simulink library "MedusaPremix"  (R2022b)
settings: Solver=VariableStepAuto  StartTime=0.0  StopTime=10.0  RelTol=1e-3
values from neighbouring files (symbols this model uses):
  PremixConfig = struct('sample_rate_in_hertz', sample_rate_in_hertz,                            'frame_size', frame_size,                            'rgain_SILENT_GAIN', rgain_SILENT_GAIN,                            'granularity', internal_granularity,                            'LR_in', LR_in, 'LR_out', LR_out,                            'CS_in', CS_in, 'CS_out', CS_out,                            'NumCenterOut' ...(+550 chars)    [MedusaPremixInit.m]
  PremixTune = MedusaPremixTuneInit(tuneFileName, headrestTuneFileName, overheadTuneFileName, MedusaParams)    [MedusaPremixInit.m]    (also in MedusaPremixTuneInit.m = load(tuneFileName))
undefined symbols (not defined in the file or in its folder): carModel, mode, MSConfig, Row
libraries: TuneVar x286, TOP x202, dspmtrx3 x146, FeaturePath x86, matrix_library x20, PooliirLib x8, Pooliir x4
(part 1 of 22)
settings Model: Creator=jk1043656  LastModifiedBy=fz1054048
settings SolverCC: AlgebraicLoopSolver=TrustRegion
settings DataIOCC: ReturnWorkspaceOutputs=off
settings DebuggingCC: UnconnectedInputMsg=warning  UnconnectedOutputMsg=warning  UnconnectedLineMsg=warning  SFMachineParentedDataDiag=warning  ArithmeticOperatorsInVariantConditions=warning
settings ModelReferenceCC: EnableRefExpFcnMdlSchedulingChecks=on
settings SFSimCC: CustomCodeUndefinedFunction=UseInterfaceOnly

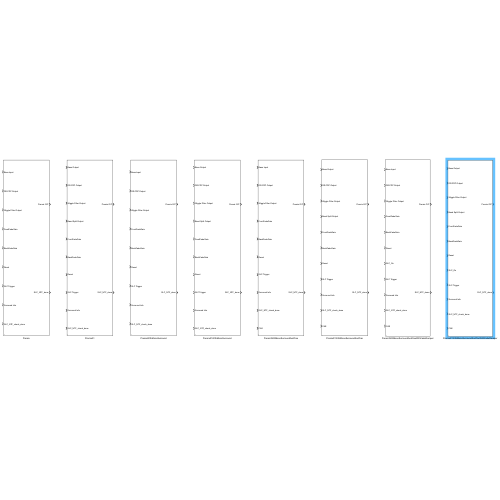
[thumbnail: Simulink's stored preview of the top-level diagram]
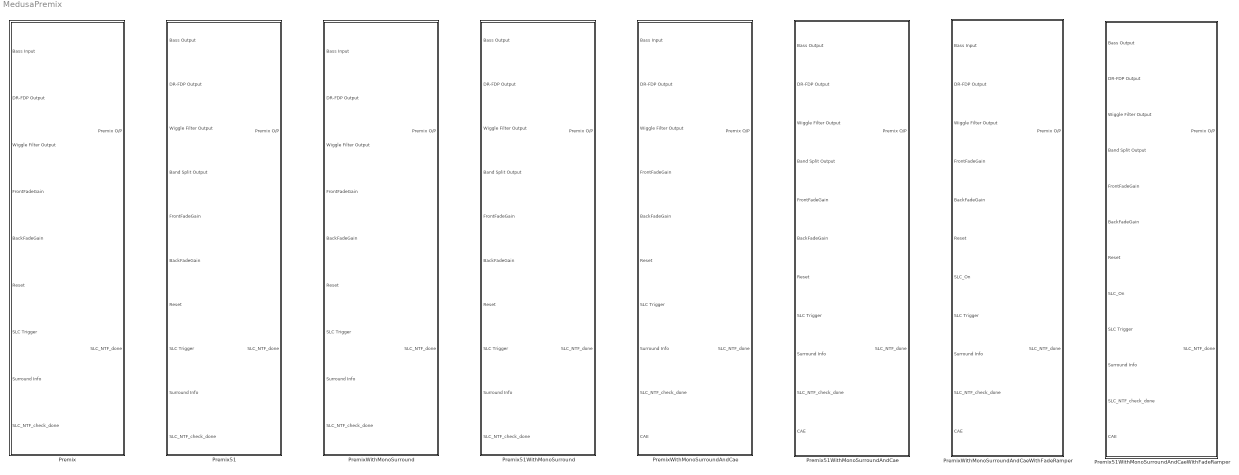
== system MedusaPremix ==
  Premix : Subsystem  mask(Medusa Premix 5H){MedusaPremixConfig=PremixConfig, MedusaPremixTune=PremixTune}
      mask prompts: MedusaPremixConfig "Config struct name:"; MedusaPremixTune "Tune struct name:"
      mask init:
      | % RTC_SIM_OBJ = RTC_SimData();
      | 
      | % MedusaConfig = generateMedusaConfig(system_definitions);
      | 
      | % Initialize model parameters
      | % MedusaPremixExampleInit(MedusaConfig);
  Premix51 : Subsystem  mask{MedusaPremixConfig=PremixConfig, MedusaPremixTune=PremixTune}
      mask prompts: MedusaPremixConfig "Config Struct Name"; MedusaPremixTune "Tune Struct Name"
      mask init:
      | % RTC_SIM_OBJ = RTC_SimData();
      | 
      | % MedusaConfig = generateMedusaConfig(system_definitions);
      | 
      | % Initialize model parameters
      | % MedusaPremixExampleInit(MedusaConfig);
  Premix51WithMonoSurround : Subsystem  mask{MedusaPremixConfig=PremixConfig, MedusaPremixTune=PremixTune, MSConfig=MSConfig}
      mask prompts: MedusaPremixConfig "Config Struct Name"; MedusaPremixTune "Tune Struct Name"; MSConfig "Mono-Surround Config"
      mask init:
      | % RTC_SIM_OBJ = RTC_SimData();
      | 
      | % MedusaConfig = generateMedusaConfig(system_definitions);
      | 
      | % Initialize model parameters
      | % MedusaPremixExampleInit(MedusaConfig);
  Premix51WithMonoSurroundAndCae : Subsystem  mask(Medusa Premix 5H){MedusaPremixConfig=PremixConfig, MedusaPremixTune=PremixTune, MSConfig=MSConfig}
      mask prompts: MedusaPremixConfig "Config struct name:"; MedusaPremixTune "Tune struct name:"; MSConfig "Mono-Surround Config:"
      mask init:
      | % RTC_SIM_OBJ = RTC_SimData();
      | 
      | % MedusaConfig = generateMedusaConfig(system_definitions);
      | 
      | % Initialize model parameters
      | % MedusaPremixExampleInit(MedusaConfig);
  Premix51WithMonoSurroundAndCaeWithFadeRamper : Subsystem  AncestorBlock=MedusaPremix/Premix 5.1 with Mono-Surround & CAE with Fade Ramper  mask(Medusa Premix 5H){MedusaPremixConfig=PremixConfig, MedusaPremixTune=PremixTune, MSConfig=MSConfig}
      mask prompts: MedusaPremixConfig "Config struct name:"; MedusaPremixTune "Tune struct name:"; MSConfig "Mono-Surround Config:"
      mask init:
      | % RTC_SIM_OBJ = RTC_SimData();
      | 
      | % MedusaConfig = generateMedusaConfig(system_definitions);
      | 
      | % Initialize model parameters
      | % MedusaPremixExampleInit(MedusaConfig);
      settings: LibrarySourceBlock=MedusaPremix/Premix 5.1 with Mono-Surround & CAE with Fade Ramper
  PremixWithMonoSurround : Subsystem  mask(Medusa Premix 5H){MedusaPremixConfig=PremixConfig, MedusaPremixTune=PremixTune, MSConfig=MSConfig}
      mask prompts: MedusaPremixConfig "Config struct name:"; MedusaPremixTune "Tune struct name:"; MSConfig "Mono-Surround Config:"
      mask init:
      | % RTC_SIM_OBJ = RTC_SimData();
      | 
      | % MedusaConfig = generateMedusaConfig(system_definitions);
      | 
      | % Initialize model parameters
      | % MedusaPremixExampleInit(MedusaConfig);
  PremixWithMonoSurroundAndCae : Subsystem  mask(Medusa Premix 5H){MedusaPremixConfig=PremixConfig, MedusaPremixTune=PremixTune, MSConfig=MSConfig}
      mask prompts: MedusaPremixConfig "Config struct name:"; MedusaPremixTune "Tune struct name:"; MSConfig "Mono-Surround Config:"
      mask init:
      | % RTC_SIM_OBJ = RTC_SimData();
      | 
      | % MedusaConfig = generateMedusaConfig(system_definitions);
      | 
      | % Initialize model parameters
      | % MedusaPremixExampleInit(MedusaConfig);
  PremixWithMonoSurroundAndCaeWithFadeRamper : Subsystem  AncestorBlock=MedusaPremix/Premix with Mono-Surround & CAE with Fade Ramper  mask(Medusa Premix 5H){MedusaPremixConfig=PremixConfig, MedusaPremixTune=PremixTune, MSConfig=MSConfig}
      mask prompts: MedusaPremixConfig "Config struct name:"; MedusaPremixTune "Tune struct name:"; MSConfig "Mono-Surround Config:"
      mask init:
      | % RTC_SIM_OBJ = RTC_SimData();
      | 
      | % MedusaConfig = generateMedusaConfig(system_definitions);
      | 
      | % Initialize model parameters
      | % MedusaPremixExampleInit(MedusaConfig);
      settings: LibrarySourceBlock=MedusaPremix/Premix with Mono-Surround & CAE with Fade Ramper

== system MedusaPremix/Premix ==
  Bass Input : Inport
  DR-FDP Output : Inport  Port=2
  Wiggle Filter Output : Inport  Port=3
  FrontFadeGain : Inport  Port=4
  BackFadeGain : Inport  Port=5
  Reset : Inport  Port=6
  SLC Trigger : Inport  Port=7
  Surround Info : Inport  Port=8
  SLC_NTF_check_done : Inport  Port=9
  Fade Inputs : Subsystem
  Fade Tuning : Subsystem
  FeaturePath : FeaturePath/FeaturePath  FeatureName=Premix  IsGroup=off  GroupNumber=-1  DeclarePackages=off  PackageNames=mode,carModel  IsToolGroup=off  TriggerInit=[145 479 260 586]
      settings: SourceProductName=Bose Talaria
  Full Mixing Matrix_Center Surround : Subsystem
  Full Mixing Matrix_Left : Subsystem
  Full Mixing Matrix_Right : Subsystem
  Function-Call Split : FunctionCallSplit  IconShape=distinctive  NumOutputPorts=3  OutputPortLayout=default
  Function-Call Split1 : FunctionCallSplit  IconShape=distinctive  NumOutputPorts=3  OutputPortLayout=default
  Input Organizer : Subsystem
  Matrix Concatenate : Concatenate  NumInputs=3  Mode=Multidimensional array  ConcatenateDimension=2
  Merge NTF_done : Subsystem
  SLC Tuning : Subsystem
  Split NTF_check_done : MATLAB Function  TreatAsAtomicUnit=on
  Premix O/P : Outport  VectorParamsAs1DForOutWhenUnconnected=off
  SLC_NTF_done : Outport  Port=2  VectorParamsAs1DForOutWhenUnconnected=off
  wires:
  Wiggle Filter Output/1 -> Input Organizer/3(WF O/P)
  Fade Inputs/2(triggerCS) -> Full Mixing Matrix_Center Surround/7(Fade Request Trigger)
  [Left_Output] -> Matrix Concatenate/2
  Function-Call Split1/2 -> Full Mixing Matrix_Center Surround/3(SLC Request Trigger)
  Function-Call Split/3 -> Full Mixing Matrix_Right/2(RST Trigger)
  Fade Inputs/5(BackFadeGain) -> Full Mixing Matrix_Left/9(Back Fade Gain), Full Mixing Matrix_Center Surround/9(Back Fade Gain), Full Mixing Matrix_Right/9(Back Fade Gain)
  Input Organizer/3(Left Channel Inputs) -> Full Mixing Matrix_Left/1(Audio Channel Inputs)
  Full Mixing Matrix_Left/1(Output) -> [Left_Output]
  Fade Inputs/1(triggerLeft) -> Full Mixing Matrix_Left/7(Fade Request Trigger)
  Full Mixing Matrix_Left/2(SLC_NTF_done) -> Merge NTF_done/1(SLC_NTF_done_Left)
  Fade Inputs/4(FrontFadeGain) -> Full Mixing Matrix_Left/8(Front Fade Gain), Full Mixing Matrix_Center Surround/8(Front Fade Gain), Full Mixing Matrix_Right/8(Front Fade Gain)
  Full Mixing Matrix_Right/2(SLC_NTF_done) -> Merge NTF_done/3(SLC_NTF_done_Right)
  Function-Call Split1/1 -> Full Mixing Matrix_Left/3(SLC Request Trigger)
  Surround Info/1 -> Full Mixing Matrix_Right/4(SLC In), Full Mixing Matrix_Center Surround/4(SLC In), Full Mixing Matrix_Left/4(SLC In)
  Split NTF_check_done/4(fcncall_AND()) -> Merge NTF_done/Trigger
  SLC Trigger/1 -> Function-Call Split1/1
  Input Organizer/1(Right Channel Inputs) -> Full Mixing Matrix_Right/1(Audio Channel Inputs)
  Function-Call Split/2 -> Full Mixing Matrix_Center Surround/2(RST Trigger)
  Input Organizer/2(CS Channel Inputs) -> Full Mixing Matrix_Center Surround/1(Audio Channel Inputs)
  Bass Input/1 -> Input Organizer/1(Bass O/P)
  Function-Call Split/1 -> Full Mixing Matrix_Left/2(RST Trigger)
  Reset/1 -> Function-Call Split/1
  Split NTF_check_done/1(fcncall_Left()) -> Full Mixing Matrix_Left/5(SLC_NTF_check_done)
  [CS_Output] -> Matrix Concatenate/1
  SLC_NTF_check_done/1 -> Split NTF_check_done/Trigger
  [Right_Output] -> Matrix Concatenate/3
  Full Mixing Matrix_Center Surround/1(Output) -> [CS_Output]
  BackFadeGain/1 -> Fade Inputs/2(BackGain)
  Split NTF_check_done/2(fcncall_CS()) -> Full Mixing Matrix_Center Surround/5(SLC_NTF_check_done)
  Matrix Concatenate/1 -> Premix O/P/1
  SLC Tuning/1(SLC Tune Out) -> Full Mixing Matrix_Left/6(SLC Tune In), Full Mixing Matrix_Center Surround/6(SLC Tune In), Full Mixing Matrix_Right/6(SLC Tune In)
  Full Mixing Matrix_Center Surround/2(SLC_NTF_done) -> Merge NTF_done/2(SLC_NTF_done_CS)
  Fade Inputs/3(triggerRight) -> Full Mixing Matrix_Right/7(Fade Request Trigger)
  Merge NTF_done/1(SLC_NTF_done) -> SLC_NTF_done/1
  FrontFadeGain/1 -> Fade Inputs/1(FrontGain)
  Split NTF_check_done/3(fcncall_Right()) -> Full Mixing Matrix_Right/5(SLC_NTF_check_done)
  Fade Tuning/1(Fade Tune Out) -> Full Mixing Matrix_Left/10(Fade Tune In), Full Mixing Matrix_Center Surround/10(Fade Tune In), Full Mixing Matrix_Right/10(Fade Tune In)
  Full Mixing Matrix_Right/1(Output) -> [Right_Output]
  DR-FDP Output/1 -> Input Organizer/2(DR-FDP O/P)
  Function-Call Split1/3 -> Full Mixing Matrix_Right/3(SLC Request Trigger)

== system MedusaPremix/Premix51 ==
  Bass Output : Inport
  DR-FDP Output : Inport  Port=2
  Wiggle Filter Output : Inport  Port=3
  Band Split Output : Inport  Port=4
  FrontFadeGain : Inport  Port=5
  BackFadeGain : Inport  Port=6
  Reset : Inport  Port=7
  SLC Trigger : Inport  Port=8
  Surround Info : Inport  Port=9
  SLC_NTF_check_done : Inport  Port=10
  Fade Inputs : Subsystem
  Fade Tuning : Subsystem
  FeaturePath : FeaturePath/FeaturePath  FeatureName=Premix  IsGroup=off  GroupNumber=-1  DeclarePackages=off  PackageNames=mode,carModel  IsToolGroup=off  TriggerInit=[575 894 690 1001]
      settings: SourceProductName=Bose Talaria
  Full Mixing Matrix_Center Surround : Subsystem
  Full Mixing Matrix_Left : Subsystem
  Full Mixing Matrix_Right : Subsystem
  Function-Call Split : FunctionCallSplit  IconShape=distinctive  NumOutputPorts=3  OutputPortLayout=default
  Function-Call Split1 : FunctionCallSplit  IconShape=distinctive  NumOutputPorts=3  OutputPortLayout=default
  Input Organizer : Subsystem
  MATLAB Function : MATLAB Function  TreatAsAtomicUnit=on
  Matrix Concatenate : Concatenate  NumInputs=3  Mode=Multidimensional array  ConcatenateDimension=2
  Merge NTF_done : Subsystem
  SLC Tuning : Subsystem
  Premix O/P : Outport  VectorParamsAs1DForOutWhenUnconnected=off
  SLC_NTF_done : Outport  Port=2  VectorParamsAs1DForOutWhenUnconnected=off
  wires:
  Full Mixing Matrix_Right/1(Output) -> [Right_Output]
  Input Organizer/2(CS Channel Inputs) -> Full Mixing Matrix_Center Surround/1(Audio Channel Inputs)
  Function-Call Split1/2 -> Full Mixing Matrix_Center Surround/3(SLC Request Trigger)
  SLC Tuning/1(SLC Tune Out) -> Full Mixing Matrix_Right/6(SLC Tune In), Full Mixing Matrix_Center Surround/6(SLC Tune In), Full Mixing Matrix_Left/6(SLC Tune In)
  [Left_Output] -> Matrix Concatenate/2
  Function-Call Split/1 -> Full Mixing Matrix_Left/2(RST Trigger)
  Bass Output/1 -> Input Organizer/1(Bass O/P)
  Input Organizer/3(Left Channel Inputs) -> Full Mixing Matrix_Left/1(Audio Channel Inputs)
  Function-Call Split1/3 -> Full Mixing Matrix_Right/3(SLC Request Trigger)
  [CS_Output] -> Matrix Concatenate/1
  Matrix Concatenate/1 -> Premix O/P/1
  DR-FDP Output/1 -> Input Organizer/2(DR-FDP O/P)
  Fade Tuning/1(Fade Tune Out) -> Full Mixing Matrix_Left/10(Fade Tune In), Full Mixing Matrix_Center Surround/10(Fade Tune In), Full Mixing Matrix_Right/10(Fade Tune In)
  Function-Call Split1/1 -> Full Mixing Matrix_Left/3(SLC Request Trigger)
  Full Mixing Matrix_Left/1(Output) -> [Left_Output]
  MATLAB Function/3(fcncall_Right()) -> Full Mixing Matrix_Right/5(SLC_NTF_check_done)
  Full Mixing Matrix_Center Surround/1(Output) -> [CS_Output]
  MATLAB Function/1(fcncall_Left()) -> Full Mixing Matrix_Left/5(SLC_NTF_check_done)
  Band Split Output/1 -> Input Organizer/4(BS O/P)
  Function-Call Split/3 -> Full Mixing Matrix_Right/2(RST Trigger)
  MATLAB Function/2(fcncall_CS()) -> Full Mixing Matrix_Center Surround/5(SLC_NTF_check_done)
  [Right_Output] -> Matrix Concatenate/3
  Function-Call Split/2 -> Full Mixing Matrix_Center Surround/2(RST Trigger)
  Merge NTF_done/1(SLC_NTF_done) -> SLC_NTF_done/1
  BackFadeGain/1 -> Fade Inputs/2(BackGain)
  Full Mixing Matrix_Center Surround/2(SLC_NTF_done) -> Merge NTF_done/2(SLC_NTF_done_CS)
  MATLAB Function/4(fcncall_AND()) -> Merge NTF_done/Trigger
  Full Mixing Matrix_Left/2(SLC_NTF_done) -> Merge NTF_done/1(SLC_NTF_done_Left)
  FrontFadeGain/1 -> Fade Inputs/1(FrontGain)
  Full Mixing Matrix_Right/2(SLC_NTF_done) -> Merge NTF_done/3(SLC_NTF_done_Right)
  Fade Inputs/1(triggerLeft) -> Full Mixing Matrix_Left/7(Fade Request Trigger)
  Surround Info/1 -> Full Mixing Matrix_Left/4(SLC In), Full Mixing Matrix_Right/4(SLC In), Full Mixing Matrix_Center Surround/4(SLC In)
  Fade Inputs/5(BackFadeGain) -> Full Mixing Matrix_Right/9(Back Fade Gain), Full Mixing Matrix_Center Surround/9(Back Fade Gain), Full Mixing Matrix_Left/9(Back Fade Gain)
  SLC Trigger/1 -> Function-Call Split1/1
  Fade Inputs/2(triggerCS) -> Full Mixing Matrix_Center Surround/7(Fade Request Trigger)
  Input Organizer/1(Right Channel Inputs) -> Full Mixing Matrix_Right/1(Audio Channel Inputs)
  Fade Inputs/3(triggerRight) -> Full Mixing Matrix_Right/7(Fade Request Trigger)
  Wiggle Filter Output/1 -> Input Organizer/3(WF O/P)
  SLC_NTF_check_done/1 -> MATLAB Function/Trigger
  Fade Inputs/4(FrontFadeGain) -> Full Mixing Matrix_Right/8(Front Fade Gain), Full Mixing Matrix_Center Surround/8(Front Fade Gain), Full Mixing Matrix_Left/8(Front Fade Gain)
  Reset/1 -> Function-Call Split/1

== system MedusaPremix/Premix51WithMonoSurround ==
  Bass Output : Inport
  DR-FDP Output : Inport  Port=2
  Wiggle Filter Output : Inport  Port=3
  Band Split Output : Inport  Port=4
  FrontFadeGain : Inport  Port=5
  BackFadeGain : Inport  Port=6
  Reset : Inport  Port=7
  SLC Trigger : Inport  Port=8
  Surround Info : Inport  Port=9
  SLC_NTF_check_done : Inport  Port=10
  CS Processing : Subsystem
  Fade Inputs : Subsystem
  Fade Tuning : Subsystem
  FeaturePath : FeaturePath/FeaturePath  FeatureName=Premix  IsGroup=off  GroupNumber=-1  IsModule=off  TriggerInit=[575 894 690 1001]
      settings: SourceProductName=Bose Talaria
  Full Mixing Matrix_Center Surround : Subsystem
  Full Mixing Matrix_Left : Subsystem
  Full Mixing Matrix_Right : Subsystem
  Function-Call Split : FunctionCallSplit  IconShape=distinctive  NumOutputPorts=3  OutputPortLayout=default
  Function-Call Split1 : FunctionCallSplit  IconShape=distinctive  NumOutputPorts=3  OutputPortLayout=default
  Input Organizer : Subsystem
  MATLAB Function : MATLAB Function  TreatAsAtomicUnit=on
  Matrix Concatenate : Concatenate  NumInputs=3  Mode=Multidimensional array  ConcatenateDimension=2
  Merge NTF_done : Subsystem
  SLC Tuning : Subsystem
  Premix O/P : Outport  VectorParamsAs1DForOutWhenUnconnected=off
  SLC_NTF_done : Outport  Port=2  VectorParamsAs1DForOutWhenUnconnected=off
  wires:
  Full Mixing Matrix_Right/1(Output) -> [Right_Output]
  Function-Call Split1/2 -> Full Mixing Matrix_Center Surround/3(SLC Request Trigger)
  SLC Tuning/1(SLC Tune Out) -> Full Mixing Matrix_Right/6(SLC Tune In), Full Mixing Matrix_Center Surround/6(SLC Tune In), Full Mixing Matrix_Left/6(SLC Tune In)
  [Left_Output] -> Matrix Concatenate/2
  Function-Call Split/1 -> Full Mixing Matrix_Left/2(RST Trigger)
  Bass Output/1 -> Input Organizer/1(Bass O/P)
  Input Organizer/3(Left Channel Inputs) -> Full Mixing Matrix_Left/1(Audio Channel Inputs)
  Function-Call Split1/3 -> Full Mixing Matrix_Right/3(SLC Request Trigger)
  [CS_Output] -> Matrix Concatenate/1
  Matrix Concatenate/1 -> Premix O/P/1
  DR-FDP Output/1 -> Input Organizer/2(DR-FDP O/P)
  Fade Tuning/1(Fade Tune Out) -> Full Mixing Matrix_Left/10(Fade Tune In), Full Mixing Matrix_Center Surround/10(Fade Tune In), Full Mixing Matrix_Right/10(Fade Tune In)
  Function-Call Split1/1 -> Full Mixing Matrix_Left/3(SLC Request Trigger)
  Full Mixing Matrix_Left/1(Output) -> [Left_Output]
  MATLAB Function/3(fcncall_Right()) -> Full Mixing Matrix_Right/5(SLC_NTF_check_done)
  Full Mixing Matrix_Center Surround/1(Output) -> [C_Output]
  MATLAB Function/1(fcncall_Left()) -> Full Mixing Matrix_Left/5(SLC_NTF_check_done)
  Band Split Output/1 -> Input Organizer/4(BS O/P)
  Function-Call Split/3 -> Full Mixing Matrix_Right/2(RST Trigger)
  MATLAB Function/2(fcncall_CS()) -> Full Mixing Matrix_Center Surround/5(SLC_NTF_check_done)
  [Right_Output] -> Matrix Concatenate/3
  Function-Call Split/2 -> Full Mixing Matrix_Center Surround/2(RST Trigger)
  Merge NTF_done/1(SLC_NTF_done) -> SLC_NTF_done/1
  BackFadeGain/1 -> Fade Inputs/2(BackGain)
  Full Mixing Matrix_Center Surround/3(SLC_NTF_done) -> Merge NTF_done/2(SLC_NTF_done_CS)
  MATLAB Function/4(fcncall_AND()) -> Merge NTF_done/Trigger
  Full Mixing Matrix_Left/2(SLC_NTF_done) -> Merge NTF_done/1(SLC_NTF_done_Left)
  FrontFadeGain/1 -> Fade Inputs/1(FrontGain)
  Full Mixing Matrix_Right/2(SLC_NTF_done) -> Merge NTF_done/3(SLC_NTF_done_Right)
  Fade Inputs/1(triggerLeft) -> Full Mixing Matrix_Left/7(Fade Request Trigger)
  Surround Info/1 -> Full Mixing Matrix_Left/4(SLC In), Full Mixing Matrix_Right/4(SLC In), Full Mixing Matrix_Center Surround/4(SLC In)
  Fade Inputs/5(BackFadeGain) -> Full Mixing Matrix_Right/9(Back Fade Gain), Full Mixing Matrix_Center Surround/9(Back Fade Gain), Full Mixing Matrix_Left/9(Back Fade Gain)
  SLC Trigger/1 -> Function-Call Split1/1
  Fade Inputs/2(triggerCS) -> Full Mixing Matrix_Center Surround/7(Fade Request Trigger)
  Input Organizer/1(Right Channel Inputs) -> Full Mixing Matrix_Right/1(Audio Channel Inputs)
  Fade Inputs/3(triggerRight) -> Full Mixing Matrix_Right/7(Fade Request Trigger)
  Wiggle Filter Output/1 -> Input Organizer/3(WF O/P)
  SLC_NTF_check_done/1 -> MATLAB Function/Trigger
  Fade Inputs/4(FrontFadeGain) -> Full Mixing Matrix_Right/8(Front Fade Gain), Full Mixing Matrix_Center Surround/8(Front Fade Gain), Full Mixing Matrix_Left/8(Front Fade Gain)
  Reset/1 -> Function-Call Split/1
  [CS_Input] -> CS Processing/2(ChanIn)
  [MS_MixCoeff] -> CS Processing/3(MixCoeff)
  [C_Output] -> CS Processing/1(COut)
  CS Processing/1(CSOut) -> [CS_Output]
  Full Mixing Matrix_Center Surround/2(MS Mixing Gains) -> [MS_MixCoeff]
  Input Organizer/2(CS Channel Inputs) -> [CS_Input], Full Mixing Matrix_Center Surround/1(Audio Channel Inputs)

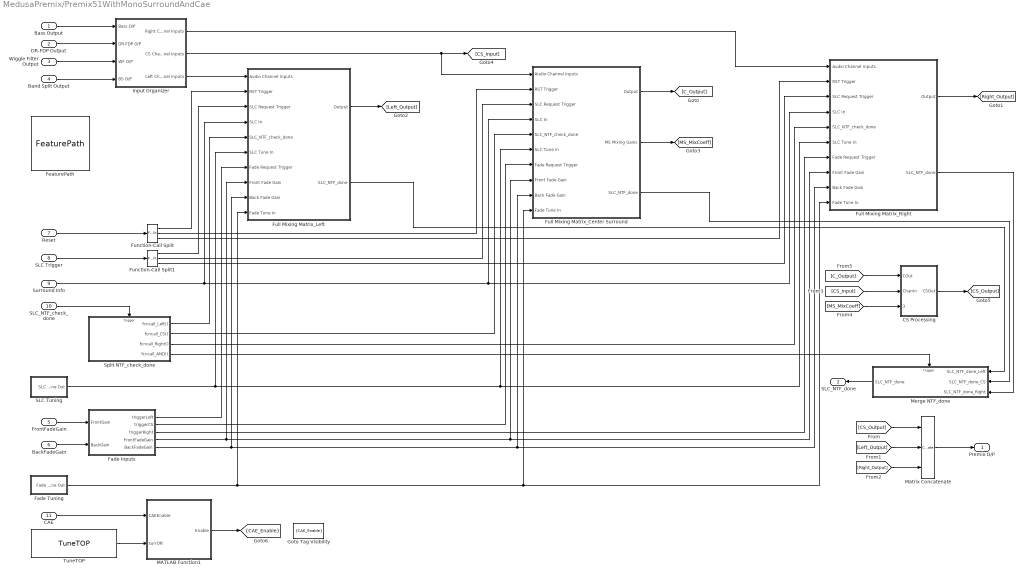
== system MedusaPremix/Premix51WithMonoSurroundAndCae ==
  Bass Output : Inport
  DR-FDP Output : Inport  Port=2
  Wiggle Filter Output : Inport  Port=3
  Band Split Output : Inport  Port=4
  FrontFadeGain : Inport  Port=5
  BackFadeGain : Inport  Port=6
  Reset : Inport  Port=7
  SLC Trigger : Inport  Port=8
  Surround Info : Inport  Port=9
  SLC_NTF_check_done : Inport  Port=10
  CAE : Inport  Port=11
  CS Processing : Subsystem
  Fade Inputs : Subsystem
  Fade Tuning : Subsystem
  FeaturePath : FeaturePath/FeaturePath  FeatureName=Premix  IsGroup=off  GroupNumber=-1  IsModule=off  TriggerInit=[145 479 260 586]
      settings: SourceProductName=Bose Talaria
  Full Mixing Matrix_Center Surround : Subsystem
  Full Mixing Matrix_Left : Subsystem
  Full Mixing Matrix_Right : Subsystem
  Function-Call Split : FunctionCallSplit  IconShape=distinctive  NumOutputPorts=3  OutputPortLayout=default
  Function-Call Split1 : FunctionCallSplit  IconShape=distinctive  NumOutputPorts=3  OutputPortLayout=default
  Goto Tag Visibility : GotoTagVisibility  GotoTag=CAE_Enable
  Input Organizer : Subsystem
  MATLAB Function1 : MATLAB Function  TreatAsAtomicUnit=on
  Matrix Concatenate : Concatenate  NumInputs=3  Mode=Multidimensional array  ConcatenateDimension=2
  Merge NTF_done : Subsystem
  SLC Tuning : Subsystem
  Split NTF_check_done : MATLAB Function  TreatAsAtomicUnit=on
  TuneTOP : TuneVar/TuneTOP  TriggerInit=[145 1297 315 1353]  TopName=SurroundON  TuneName=SurroundON  DataType=single  TunabilityNumber=1  MinValue=[]  MaxValue=[]  BankNumber=0  PreOverlay=false  PostOverlay=false  UseSameName=on  MaskValue=2
      settings: SourceProductName=Bose Talaria
  Premix O/P : Outport  VectorParamsAs1DForOutWhenUnconnected=off
  SLC_NTF_done : Outport  Port=2  VectorParamsAs1DForOutWhenUnconnected=off
  tag scope: CAE_Enable=scoped
  wires:
  [CS_Input] -> CS Processing/2(ChanIn)
  [MS_MixCoeff] -> CS Processing/3(MixCoeff)
  CS Processing/1(CSOut) -> [CS_Output]
  [C_Output] -> CS Processing/1(COut)
  Input Organizer/2(CS Channel Inputs) -> Full Mixing Matrix_Center Surround/1(Audio Channel Inputs), [CS_Input]
  Full Mixing Matrix_Center Surround/2(MS Mixing Gains) -> [MS_MixCoeff]
  Function-Call Split1/3 -> Full Mixing Matrix_Right/3(SLC Request Trigger)
  Full Mixing Matrix_Right/1(Output) -> [Right_Output]
  Fade Tuning/1(Fade Tune Out) -> Full Mixing Matrix_Right/10(Fade Tune In), Full Mixing Matrix_Center Surround/10(Fade Tune In), Full Mixing Matrix_Left/10(Fade Tune In)
  Split NTF_check_done/3(fcncall_Right()) -> Full Mixing Matrix_Right/5(SLC_NTF_check_done)
  FrontFadeGain/1 -> Fade Inputs/1(FrontGain)
  Merge NTF_done/1(SLC_NTF_done) -> SLC_NTF_done/1
  Fade Inputs/3(triggerRight) -> Full Mixing Matrix_Right/7(Fade Request Trigger)
  Full Mixing Matrix_Center Surround/3(SLC_NTF_done) -> Merge NTF_done/2(SLC_NTF_done_CS)
  SLC Tuning/1(SLC Tune Out) -> Full Mixing Matrix_Right/6(SLC Tune In), Full Mixing Matrix_Center Surround/6(SLC Tune In), Full Mixing Matrix_Left/6(SLC Tune In)
  Matrix Concatenate/1 -> Premix O/P/1
  Split NTF_check_done/2(fcncall_CS()) -> Full Mixing Matrix_Center Surround/5(SLC_NTF_check_done)
  BackFadeGain/1 -> Fade Inputs/2(BackGain)
  Full Mixing Matrix_Center Surround/1(Output) -> [C_Output]
  [Right_Output] -> Matrix Concatenate/3
  SLC_NTF_check_done/1 -> Split NTF_check_done/Trigger
  [CS_Output] -> Matrix Concatenate/1
  Split NTF_check_done/1(fcncall_Left()) -> Full Mixing Matrix_Left/5(SLC_NTF_check_done)
  Reset/1 -> Function-Call Split/1
  Function-Call Split/1 -> Full Mixing Matrix_Left/2(RST Trigger)
  Function-Call Split/2 -> Full Mixing Matrix_Center Surround/2(RST Trigger)
  Input Organizer/1(Right Channel Inputs) -> Full Mixing Matrix_Right/1(Audio Channel Inputs)
  SLC Trigger/1 -> Function-Call Split1/1
  Split NTF_check_done/4(fcncall_AND()) -> Merge NTF_done/Trigger
  Surround Info/1 -> Full Mixing Matrix_Left/4(SLC In), Full Mixing Matrix_Center Surround/4(SLC In), Full Mixing Matrix_Right/4(SLC In)
  Function-Call Split1/1 -> Full Mixing Matrix_Left/3(SLC Request Trigger)
  Full Mixing Matrix_Right/2(SLC_NTF_done) -> Merge NTF_done/3(SLC_NTF_done_Right)
  Fade Inputs/4(FrontFadeGain) -> Full Mixing Matrix_Right/8(Front Fade Gain), Full Mixing Matrix_Center Surround/8(Front Fade Gain), Full Mixing Matrix_Left/8(Front Fade Gain)
  Full Mixing Matrix_Left/2(SLC_NTF_done) -> Merge NTF_done/1(SLC_NTF_done_Left)
  Fade Inputs/1(triggerLeft) -> Full Mixing Matrix_Left/7(Fade Request Trigger)
  Full Mixing Matrix_Left/1(Output) -> [Left_Output]
  Input Organizer/3(Left Channel Inputs) -> Full Mixing Matrix_Left/1(Audio Channel Inputs)
  Fade Inputs/5(BackFadeGain) -> Full Mixing Matrix_Right/9(Back Fade Gain), Full Mixing Matrix_Center Surround/9(Back Fade Gain), Full Mixing Matrix_Left/9(Back Fade Gain)
  Function-Call Split/3 -> Full Mixing Matrix_Right/2(RST Trigger)
  Function-Call Split1/2 -> Full Mixing Matrix_Center Surround/3(SLC Request Trigger)
  [Left_Output] -> Matrix Concatenate/2
  Fade Inputs/2(triggerCS) -> Full Mixing Matrix_Center Surround/7(Fade Request Trigger)
  Wiggle Filter Output/1 -> Input Organizer/3(WF O/P)
  DR-FDP Output/1 -> Input Organizer/2(DR-FDP O/P)
  Band Split Output/1 -> Input Organizer/4(BS O/P)
  Bass Output/1 -> Input Organizer/1(Bass O/P)
  CAE/1 -> MATLAB Function1/1(CAEEnable)
  TuneTOP/1 -> MATLAB Function1/2(surrON)
  MATLAB Function1/1(Enable) -> [CAE_Enable]

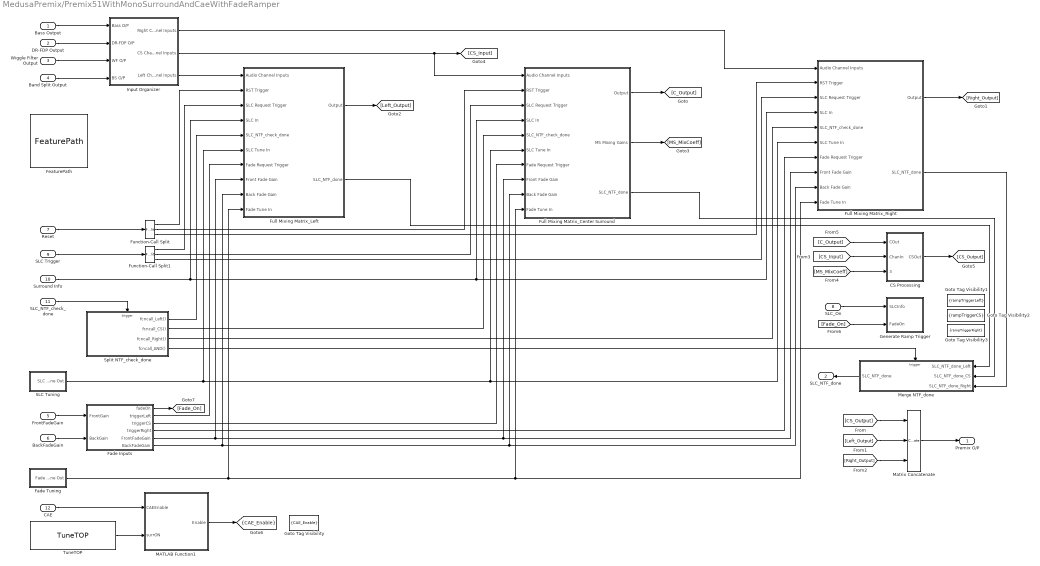
== system MedusaPremix/Premix51WithMonoSurroundAndCaeWithFadeRamper ==
  Bass Output : Inport
  DR-FDP Output : Inport  Port=2
  Wiggle Filter Output : Inport  Port=3
  Band Split Output : Inport  Port=4
  FrontFadeGain : Inport  Port=5
  BackFadeGain : Inport  Port=6
  Reset : Inport  Port=7
  SLC_On : Inport  Port=8
  SLC Trigger : Inport  Port=9
  Surround Info : Inport  Port=10
  SLC_NTF_check_done : Inport  Port=11
  CAE : Inport  Port=12
  CS Processing : Subsystem
  Fade Inputs : Subsystem
  Fade Tuning : Subsystem
  FeaturePath : FeaturePath/FeaturePath  FeatureName=Premix  IsGroup=off  GroupNumber=-1  IsModule=off  TriggerInit=[145 479 260 586]
      settings: SourceProductName=Bose Talaria
  Full Mixing Matrix_Center Surround : Subsystem
  Full Mixing Matrix_Left : Subsystem
  Full Mixing Matrix_Right : Subsystem
  Function-Call Split : FunctionCallSplit  IconShape=distinctive  NumOutputPorts=3  OutputPortLayout=default
  Function-Call Split1 : FunctionCallSplit  IconShape=distinctive  NumOutputPorts=3  OutputPortLayout=default
  Generate Ramp Trigger : Subsystem
  Goto Tag Visibility : GotoTagVisibility  GotoTag=CAE_Enable
  Goto Tag Visibility1 : GotoTagVisibility  GotoTag=rampTriggerLeft
  Goto Tag Visibility2 : GotoTagVisibility  GotoTag=rampTriggerCS
  Goto Tag Visibility3 : GotoTagVisibility  GotoTag=rampTriggerRight
  Input Organizer : Subsystem
  MATLAB Function1 : MATLAB Function  TreatAsAtomicUnit=on
  Matrix Concatenate : Concatenate  NumInputs=3  Mode=Multidimensional array  ConcatenateDimension=2
  Merge NTF_done : Subsystem
  SLC Tuning : Subsystem
  Split NTF_check_done : MATLAB Function  TreatAsAtomicUnit=on
  TuneTOP : TuneVar/TuneTOP  TriggerInit=[145 1297 315 1353]  TopName=SurroundON  TuneName=SurroundON  DataType=single  TunabilityNumber=1  MinValue=[]  MaxValue=[]  BankNumber=0  PreOverlay=false  PostOverlay=false  UseSameName=on  MaskValue=2
      settings: SourceProductName=Bose Talaria
  Premix O/P : Outport  VectorParamsAs1DForOutWhenUnconnected=off
  SLC_NTF_done : Outport  Port=2  VectorParamsAs1DForOutWhenUnconnected=off
  tag scope: CAE_Enable=scoped
  wires:
  [CS_Input] -> CS Processing/2(ChanIn)
  [MS_MixCoeff] -> CS Processing/3(MixCoeff)
  CS Processing/1(CSOut) -> [CS_Output]
  [C_Output] -> CS Processing/1(COut)
  Input Organizer/2(CS Channel Inputs) -> Full Mixing Matrix_Center Surround/1(Audio Channel Inputs), [CS_Input]
  Full Mixing Matrix_Center Surround/2(MS Mixing Gains) -> [MS_MixCoeff]
  Function-Call Split1/3 -> Full Mixing Matrix_Right/3(SLC Request Trigger)
  Full Mixing Matrix_Right/1(Output) -> [Right_Output]
  Fade Tuning/1(Fade Tune Out) -> Full Mixing Matrix_Right/10(Fade Tune In), Full Mixing Matrix_Center Surround/10(Fade Tune In), Full Mixing Matrix_Left/10(Fade Tune In)
  Split NTF_check_done/3(fcncall_Right()) -> Full Mixing Matrix_Right/5(SLC_NTF_check_done)
  FrontFadeGain/1 -> Fade Inputs/1(FrontGain)
  Merge NTF_done/1(SLC_NTF_done) -> SLC_NTF_done/1
  Fade Inputs/4(triggerRight) -> Full Mixing Matrix_Right/7(Fade Request Trigger)
  Full Mixing Matrix_Center Surround/3(SLC_NTF_done) -> Merge NTF_done/2(SLC_NTF_done_CS)
  SLC Tuning/1(SLC Tune Out) -> Full Mixing Matrix_Right/6(SLC Tune In), Full Mixing Matrix_Center Surround/6(SLC Tune In), Full Mixing Matrix_Left/6(SLC Tune In)
  Matrix Concatenate/1 -> Premix O/P/1
  Split NTF_check_done/2(fcncall_CS()) -> Full Mixing Matrix_Center Surround/5(SLC_NTF_check_done)
  BackFadeGain/1 -> Fade Inputs/2(BackGain)
  Full Mixing Matrix_Center Surround/1(Output) -> [C_Output]
  [Right_Output] -> Matrix Concatenate/3
  SLC_NTF_check_done/1 -> Split NTF_check_done/Trigger
  [CS_Output] -> Matrix Concatenate/1
  Split NTF_check_done/1(fcncall_Left()) -> Full Mixing Matrix_Left/5(SLC_NTF_check_done)
  Reset/1 -> Function-Call Split/1
  Function-Call Split/1 -> Full Mixing Matrix_Left/2(RST Trigger)
  Function-Call Split/2 -> Full Mixing Matrix_Center Surround/2(RST Trigger)
  Input Organizer/1(Right Channel Inputs) -> Full Mixing Matrix_Right/1(Audio Channel Inputs)
  SLC Trigger/1 -> Function-Call Split1/1
  Split NTF_check_done/4(fcncall_AND()) -> Merge NTF_done/Trigger
  Surround Info/1 -> Full Mixing Matrix_Right/4(SLC In), Full Mixing Matrix_Center Surround/4(SLC In), Full Mixing Matrix_Left/4(SLC In)
  Function-Call Split1/1 -> Full Mixing Matrix_Left/3(SLC Request Trigger)
  Full Mixing Matrix_Right/2(SLC_NTF_done) -> Merge NTF_done/3(SLC_NTF_done_Right)
  Fade Inputs/5(FrontFadeGain) -> Full Mixing Matrix_Center Surround/8(Front Fade Gain), Full Mixing Matrix_Right/8(Front Fade Gain), Full Mixing Matrix_Left/8(Front Fade Gain)
  Full Mixing Matrix_Left/2(SLC_NTF_done) -> Merge NTF_done/1(SLC_NTF_done_Left)
  Fade Inputs/2(triggerLeft) -> Full Mixing Matrix_Left/7(Fade Request Trigger)
  Full Mixing Matrix_Left/1(Output) -> [Left_Output]
  Input Organizer/3(Left Channel Inputs) -> Full Mixing Matrix_Left/1(Audio Channel Inputs)
  Fade Inputs/6(BackFadeGain) -> Full Mixing Matrix_Center Surround/9(Back Fade Gain), Full Mixing Matrix_Right/9(Back Fade Gain), Full Mixing Matrix_Left/9(Back Fade Gain)
  Function-Call Split/3 -> Full Mixing Matrix_Right/2(RST Trigger)
  Function-Call Split1/2 -> Full Mixing Matrix_Center Surround/3(SLC Request Trigger)
  [Left_Output] -> Matrix Concatenate/2
  Fade Inputs/3(triggerCS) -> Full Mixing Matrix_Center Surround/7(Fade Request Trigger)
  Fade Inputs/1(fadeOn) -> [Fade_On]
  SLC_On/1 -> Generate Ramp Trigger/1(SLCInfo)
  [Fade_On] -> Generate Ramp Trigger/2(FadeOn)
  Band Split Output/1 -> Input Organizer/4(BS O/P)
  Bass Output/1 -> Input Organizer/1(Bass O/P)
  Wiggle Filter Output/1 -> Input Organizer/3(WF O/P)
  DR-FDP Output/1 -> Input Organizer/2(DR-FDP O/P)
  MATLAB Function1/1(Enable) -> [CAE_Enable]
  CAE/1 -> MATLAB Function1/1(CAEEnable)
  TuneTOP/1 -> MATLAB Function1/2(surrON)

== system MedusaPremix/PremixWithMonoSurround ==
  Bass Input : Inport
  DR-FDP Output : Inport  Port=2
  Wiggle Filter Output : Inport  Port=3
  FrontFadeGain : Inport  Port=4
  BackFadeGain : Inport  Port=5
  Reset : Inport  Port=6
  SLC Trigger : Inport  Port=7
  Surround Info : Inport  Port=8
  SLC_NTF_check_done : Inport  Port=9
  CS Processing : Subsystem
  Fade Inputs : Subsystem
  Fade Tuning : Subsystem
  FeaturePath : FeaturePath/FeaturePath  FeatureName=Premix  IsGroup=off  GroupNumber=-1  DeclarePackages=off  PackageNames=mode,carModel  IsToolGroup=off  TriggerInit=[145 479 260 586]
      settings: SourceProductName=Bose Talaria
  Full Mixing Matrix_Center Surround : Subsystem
  Full Mixing Matrix_Left : Subsystem
  Full Mixing Matrix_Right : Subsystem
  Function-Call Split : FunctionCallSplit  IconShape=distinctive  NumOutputPorts=3  OutputPortLayout=default
  Function-Call Split1 : FunctionCallSplit  IconShape=distinctive  NumOutputPorts=3  OutputPortLayout=default
  Input Organizer : Subsystem
  Matrix Concatenate : Concatenate  NumInputs=3  Mode=Multidimensional array  ConcatenateDimension=2
  Merge NTF_done : Subsystem
  SLC Tuning : Subsystem
  Split NTF_check_done : MATLAB Function  TreatAsAtomicUnit=on
  Premix O/P : Outport  VectorParamsAs1DForOutWhenUnconnected=off
  SLC_NTF_done : Outport  Port=2  VectorParamsAs1DForOutWhenUnconnected=off
  wires:
  Function-Call Split1/3 -> Full Mixing Matrix_Right/3(SLC Request Trigger)
  DR-FDP Output/1 -> Input Organizer/2(DR-FDP O/P)
  Full Mixing Matrix_Right/1(Output) -> [Right_Output]
  Fade Tuning/1(Fade Tune Out) -> Full Mixing Matrix_Right/10(Fade Tune In), Full Mixing Matrix_Center Surround/10(Fade Tune In), Full Mixing Matrix_Left/10(Fade Tune In)
  Split NTF_check_done/3(fcncall_Right()) -> Full Mixing Matrix_Right/5(SLC_NTF_check_done)
  FrontFadeGain/1 -> Fade Inputs/1(FrontGain)
  Merge NTF_done/1(SLC_NTF_done) -> SLC_NTF_done/1
  Fade Inputs/3(triggerRight) -> Full Mixing Matrix_Right/7(Fade Request Trigger)
  Full Mixing Matrix_Center Surround/3(SLC_NTF_done) -> Merge NTF_done/2(SLC_NTF_done_CS)
  SLC Tuning/1(SLC Tune Out) -> Full Mixing Matrix_Right/6(SLC Tune In), Full Mixing Matrix_Center Surround/6(SLC Tune In), Full Mixing Matrix_Left/6(SLC Tune In)
  Matrix Concatenate/1 -> Premix O/P/1
  Split NTF_check_done/2(fcncall_CS()) -> Full Mixing Matrix_Center Surround/5(SLC_NTF_check_done)
  BackFadeGain/1 -> Fade Inputs/2(BackGain)
  Full Mixing Matrix_Center Surround/1(Output) -> [C_Output]
  [Right_Output] -> Matrix Concatenate/3
  SLC_NTF_check_done/1 -> Split NTF_check_done/Trigger
  [CS_Output] -> Matrix Concatenate/1
  Split NTF_check_done/1(fcncall_Left()) -> Full Mixing Matrix_Left/5(SLC_NTF_check_done)
  Reset/1 -> Function-Call Split/1
  Function-Call Split/1 -> Full Mixing Matrix_Left/2(RST Trigger)
  Bass Input/1 -> Input Organizer/1(Bass O/P)
  Input Organizer/2(CS Channel Inputs) -> [CS_Input], Full Mixing Matrix_Center Surround/1(Audio Channel Inputs)
  Function-Call Split/2 -> Full Mixing Matrix_Center Surround/2(RST Trigger)
  Input Organizer/1(Right Channel Inputs) -> Full Mixing Matrix_Right/1(Audio Channel Inputs)
  SLC Trigger/1 -> Function-Call Split1/1
  Split NTF_check_done/4(fcncall_AND()) -> Merge NTF_done/Trigger
  Surround Info/1 -> Full Mixing Matrix_Left/4(SLC In), Full Mixing Matrix_Center Surround/4(SLC In), Full Mixing Matrix_Right/4(SLC In)
  Function-Call Split1/1 -> Full Mixing Matrix_Left/3(SLC Request Trigger)
  Full Mixing Matrix_Right/2(SLC_NTF_done) -> Merge NTF_done/3(SLC_NTF_done_Right)
  Fade Inputs/4(FrontFadeGain) -> Full Mixing Matrix_Right/8(Front Fade Gain), Full Mixing Matrix_Center Surround/8(Front Fade Gain), Full Mixing Matrix_Left/8(Front Fade Gain)
  Full Mixing Matrix_Left/2(SLC_NTF_done) -> Merge NTF_done/1(SLC_NTF_done_Left)
  Fade Inputs/1(triggerLeft) -> Full Mixing Matrix_Left/7(Fade Request Trigger)
  Full Mixing Matrix_Left/1(Output) -> [Left_Output]
  Input Organizer/3(Left Channel Inputs) -> Full Mixing Matrix_Left/1(Audio Channel Inputs)
  Fade Inputs/5(BackFadeGain) -> Full Mixing Matrix_Right/9(Back Fade Gain), Full Mixing Matrix_Center Surround/9(Back Fade Gain), Full Mixing Matrix_Left/9(Back Fade Gain)
  Function-Call Split/3 -> Full Mixing Matrix_Right/2(RST Trigger)
  Function-Call Split1/2 -> Full Mixing Matrix_Center Surround/3(SLC Request Trigger)
  [Left_Output] -> Matrix Concatenate/2
  Fade Inputs/2(triggerCS) -> Full Mixing Matrix_Center Surround/7(Fade Request Trigger)
  Wiggle Filter Output/1 -> Input Organizer/3(WF O/P)
  Full Mixing Matrix_Center Surround/2(MS Mixing Gains) -> [MS_MixCoeff]
  [C_Output] -> CS Processing/1(COut)
  CS Processing/1(CSOut) -> [CS_Output]
  [MS_MixCoeff] -> CS Processing/3(MixCoeff)
  [CS_Input] -> CS Processing/2(ChanIn)

== system MedusaPremix/PremixWithMonoSurroundAndCae ==
  Bass Input : Inport
  DR-FDP Output : Inport  Port=2
  Wiggle Filter Output : Inport  Port=3
  FrontFadeGain : Inport  Port=4
  BackFadeGain : Inport  Port=5
  Reset : Inport  Port=6
  SLC Trigger : Inport  Port=7
  Surround Info : Inport  Port=8
  SLC_NTF_check_done : Inport  Port=9
  CAE : Inport  Port=10
  CS Processing : Subsystem
  Fade Inputs : Subsystem
  Fade Tuning : Subsystem
  FeaturePath : FeaturePath/FeaturePath  FeatureName=Premix  IsGroup=off  GroupNumber=-1  IsModule=off  TriggerInit=[145 479 260 586]
      settings: SourceProductName=Bose Talaria
  Full Mixing Matrix_Center Surround : Subsystem
  Full Mixing Matrix_Left : Subsystem
  Full Mixing Matrix_Right : Subsystem
  Function-Call Split : FunctionCallSplit  IconShape=distinctive  NumOutputPorts=3  OutputPortLayout=default
  Function-Call Split1 : FunctionCallSplit  IconShape=distinctive  NumOutputPorts=3  OutputPortLayout=default
  Goto Tag Visibility : GotoTagVisibility  GotoTag=CAE_Enable
  Input Organizer : Subsystem
  Matrix Concatenate : Concatenate  NumInputs=3  Mode=Multidimensional array  ConcatenateDimension=2
  Merge NTF_done : Subsystem
  SLC Tuning : Subsystem
  Split NTF_check_done : MATLAB Function  TreatAsAtomicUnit=on
  Premix O/P : Outport  VectorParamsAs1DForOutWhenUnconnected=off
  SLC_NTF_done : Outport  Port=2  VectorParamsAs1DForOutWhenUnconnected=off
  tag scope: CAE_Enable=scoped
  wires:
  [CS_Input] -> CS Processing/2(ChanIn)
  [MS_MixCoeff] -> CS Processing/3(MixCoeff)
  CS Processing/1(CSOut) -> [CS_Output]
  [C_Output] -> CS Processing/1(COut)
  Input Organizer/2(CS Channel Inputs) -> Full Mixing Matrix_Center Surround/1(Audio Channel Inputs), [CS_Input]
  Full Mixing Matrix_Center Surround/2(MS Mixing Gains) -> [MS_MixCoeff]
  CAE/1 -> [CAE_Enable]
  Function-Call Split1/3 -> Full Mixing Matrix_Right/3(SLC Request Trigger)
  DR-FDP Output/1 -> Input Organizer/2(DR-FDP O/P)
  Full Mixing Matrix_Right/1(Output) -> [Right_Output]
  Fade Tuning/1(Fade Tune Out) -> Full Mixing Matrix_Right/10(Fade Tune In), Full Mixing Matrix_Center Surround/10(Fade Tune In), Full Mixing Matrix_Left/10(Fade Tune In)
  Split NTF_check_done/3(fcncall_Right()) -> Full Mixing Matrix_Right/5(SLC_NTF_check_done)
  FrontFadeGain/1 -> Fade Inputs/1(FrontGain)
  Merge NTF_done/1(SLC_NTF_done) -> SLC_NTF_done/1
  Fade Inputs/3(triggerRight) -> Full Mixing Matrix_Right/7(Fade Request Trigger)
  Full Mixing Matrix_Center Surround/3(SLC_NTF_done) -> Merge NTF_done/2(SLC_NTF_done_CS)
  SLC Tuning/1(SLC Tune Out) -> Full Mixing Matrix_Right/6(SLC Tune In), Full Mixing Matrix_Center Surround/6(SLC Tune In), Full Mixing Matrix_Left/6(SLC Tune In)
  Matrix Concatenate/1 -> Premix O/P/1
  Split NTF_check_done/2(fcncall_CS()) -> Full Mixing Matrix_Center Surround/5(SLC_NTF_check_done)
  BackFadeGain/1 -> Fade Inputs/2(BackGain)
  Full Mixing Matrix_Center Surround/1(Output) -> [C_Output]
  [Right_Output] -> Matrix Concatenate/3
  SLC_NTF_check_done/1 -> Split NTF_check_done/Trigger
  [CS_Output] -> Matrix Concatenate/1
  Split NTF_check_done/1(fcncall_Left()) -> Full Mixing Matrix_Left/5(SLC_NTF_check_done)
  Reset/1 -> Function-Call Split/1
  Function-Call Split/1 -> Full Mixing Matrix_Left/2(RST Trigger)
  Bass Input/1 -> Input Organizer/1(Bass O/P)
  Function-Call Split/2 -> Full Mixing Matrix_Center Surround/2(RST Trigger)
  Input Organizer/1(Right Channel Inputs) -> Full Mixing Matrix_Right/1(Audio Channel Inputs)
  SLC Trigger/1 -> Function-Call Split1/1
  Split NTF_check_done/4(fcncall_AND()) -> Merge NTF_done/Trigger
  Surround Info/1 -> Full Mixing Matrix_Left/4(SLC In), Full Mixing Matrix_Center Surround/4(SLC In), Full Mixing Matrix_Right/4(SLC In)
  Function-Call Split1/1 -> Full Mixing Matrix_Left/3(SLC Request Trigger)
  Full Mixing Matrix_Right/2(SLC_NTF_done) -> Merge NTF_done/3(SLC_NTF_done_Right)
  Fade Inputs/4(FrontFadeGain) -> Full Mixing Matrix_Right/8(Front Fade Gain), Full Mixing Matrix_Center Surround/8(Front Fade Gain), Full Mixing Matrix_Left/8(Front Fade Gain)
  Full Mixing Matrix_Left/2(SLC_NTF_done) -> Merge NTF_done/1(SLC_NTF_done_Left)
  Fade Inputs/1(triggerLeft) -> Full Mixing Matrix_Left/7(Fade Request Trigger)
  Full Mixing Matrix_Left/1(Output) -> [Left_Output]
  Input Organizer/3(Left Channel Inputs) -> Full Mixing Matrix_Left/1(Audio Channel Inputs)
  Fade Inputs/5(BackFadeGain) -> Full Mixing Matrix_Right/9(Back Fade Gain), Full Mixing Matrix_Center Surround/9(Back Fade Gain), Full Mixing Matrix_Left/9(Back Fade Gain)
  Function-Call Split/3 -> Full Mixing Matrix_Right/2(RST Trigger)
  Function-Call Split1/2 -> Full Mixing Matrix_Center Surround/3(SLC Request Trigger)
  [Left_Output] -> Matrix Concatenate/2
  Fade Inputs/2(triggerCS) -> Full Mixing Matrix_Center Surround/7(Fade Request Trigger)
  Wiggle Filter Output/1 -> Input Organizer/3(WF O/P)

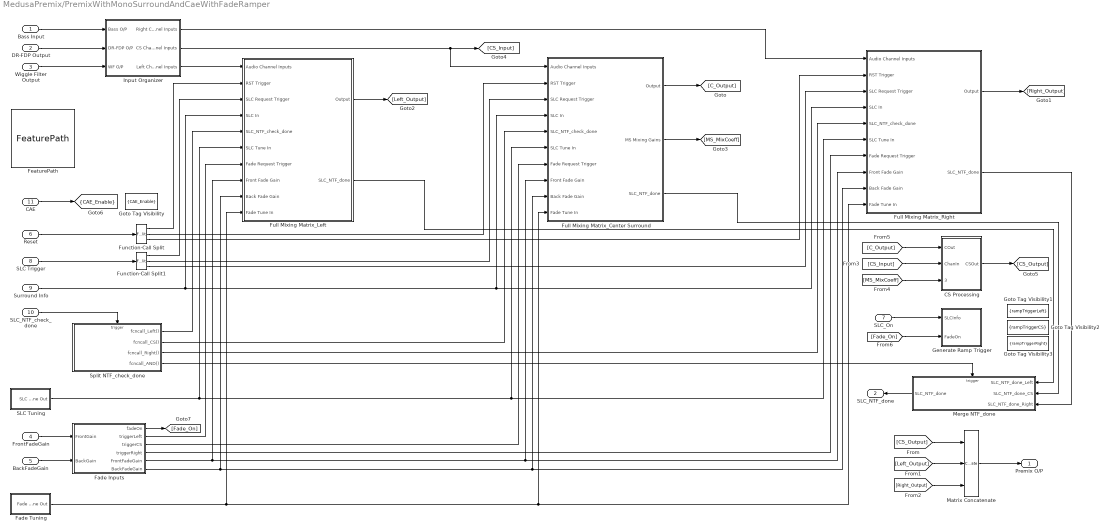
== system MedusaPremix/PremixWithMonoSurroundAndCaeWithFadeRamper ==
  Bass Input : Inport
  DR-FDP Output : Inport  Port=2
  Wiggle Filter Output : Inport  Port=3
  FrontFadeGain : Inport  Port=4
  BackFadeGain : Inport  Port=5
  Reset : Inport  Port=6
  SLC_On : Inport  Port=7
  SLC Trigger : Inport  Port=8
  Surround Info : Inport  Port=9
  SLC_NTF_check_done : Inport  Port=10
  CAE : Inport  Port=11
  CS Processing : Subsystem
  Fade Inputs : Subsystem
  Fade Tuning : Subsystem
  FeaturePath : FeaturePath/FeaturePath  FeatureName=Premix  IsGroup=off  GroupNumber=-1  IsModule=off  TriggerInit=[145 479 260 586]
      settings: SourceProductName=Bose Talaria
  Full Mixing Matrix_Center Surround : Subsystem
  Full Mixing Matrix_Left : Subsystem
  Full Mixing Matrix_Right : Subsystem
  Function-Call Split : FunctionCallSplit  IconShape=distinctive  NumOutputPorts=3  OutputPortLayout=default
  Function-Call Split1 : FunctionCallSplit  IconShape=distinctive  NumOutputPorts=3  OutputPortLayout=default
  Generate Ramp Trigger : Subsystem
  Goto Tag Visibility : GotoTagVisibility  GotoTag=CAE_Enable
  Goto Tag Visibility1 : GotoTagVisibility  GotoTag=rampTriggerLeft
  Goto Tag Visibility2 : GotoTagVisibility  GotoTag=rampTriggerCS
  Goto Tag Visibility3 : GotoTagVisibility  GotoTag=rampTriggerRight
  Input Organizer : Subsystem
  Matrix Concatenate : Concatenate  NumInputs=3  Mode=Multidimensional array  ConcatenateDimension=2
  Merge NTF_done : Subsystem
  SLC Tuning : Subsystem
  Split NTF_check_done : MATLAB Function  TreatAsAtomicUnit=on
  Premix O/P : Outport  VectorParamsAs1DForOutWhenUnconnected=off
  SLC_NTF_done : Outport  Port=2  VectorParamsAs1DForOutWhenUnconnected=off
  tag scope: CAE_Enable=scoped
  wires:
  [Fade_On] -> Generate Ramp Trigger/2(FadeOn)
  SLC_On/1 -> Generate Ramp Trigger/1(SLCInfo)
  Fade Inputs/1(fadeOn) -> [Fade_On]
  Wiggle Filter Output/1 -> Input Organizer/3(WF O/P)
  Fade Inputs/3(triggerCS) -> Full Mixing Matrix_Center Surround/7(Fade Request Trigger)
  [Left_Output] -> Matrix Concatenate/2
  Function-Call Split1/2 -> Full Mixing Matrix_Center Surround/3(SLC Request Trigger)
  Function-Call Split/3 -> Full Mixing Matrix_Right/2(RST Trigger)
  Fade Inputs/6(BackFadeGain) -> Full Mixing Matrix_Left/9(Back Fade Gain), Full Mixing Matrix_Right/9(Back Fade Gain), Full Mixing Matrix_Center Surround/9(Back Fade Gain)
  Input Organizer/3(Left Channel Inputs) -> Full Mixing Matrix_Left/1(Audio Channel Inputs)
  Full Mixing Matrix_Left/1(Output) -> [Left_Output]
  Fade Inputs/2(triggerLeft) -> Full Mixing Matrix_Left/7(Fade Request Trigger)
  Full Mixing Matrix_Left/2(SLC_NTF_done) -> Merge NTF_done/1(SLC_NTF_done_Left)
  Fade Inputs/5(FrontFadeGain) -> Full Mixing Matrix_Left/8(Front Fade Gain), Full Mixing Matrix_Right/8(Front Fade Gain), Full Mixing Matrix_Center Surround/8(Front Fade Gain)
  Full Mixing Matrix_Right/2(SLC_NTF_done) -> Merge NTF_done/3(SLC_NTF_done_Right)
  Function-Call Split1/1 -> Full Mixing Matrix_Left/3(SLC Request Trigger)
  Surround Info/1 -> Full Mixing Matrix_Left/4(SLC In), Full Mixing Matrix_Center Surround/4(SLC In), Full Mixing Matrix_Right/4(SLC In)
  Split NTF_check_done/4(fcncall_AND()) -> Merge NTF_done/Trigger
  SLC Trigger/1 -> Function-Call Split1/1
  Input Organizer/1(Right Channel Inputs) -> Full Mixing Matrix_Right/1(Audio Channel Inputs)
  Function-Call Split/2 -> Full Mixing Matrix_Center Surround/2(RST Trigger)
  Bass Input/1 -> Input Organizer/1(Bass O/P)
  Function-Call Split/1 -> Full Mixing Matrix_Left/2(RST Trigger)
  Reset/1 -> Function-Call Split/1
  Split NTF_check_done/1(fcncall_Left()) -> Full Mixing Matrix_Left/5(SLC_NTF_check_done)
  [CS_Output] -> Matrix Concatenate/1
  SLC_NTF_check_done/1 -> Split NTF_check_done/Trigger
  [Right_Output] -> Matrix Concatenate/3
  Full Mixing Matrix_Center Surround/1(Output) -> [C_Output]
  BackFadeGain/1 -> Fade Inputs/2(BackGain)
  Split NTF_check_done/2(fcncall_CS()) -> Full Mixing Matrix_Center Surround/5(SLC_NTF_check_done)
  Matrix Concatenate/1 -> Premix O/P/1
  SLC Tuning/1(SLC Tune Out) -> Full Mixing Matrix_Left/6(SLC Tune In), Full Mixing Matrix_Center Surround/6(SLC Tune In), Full Mixing Matrix_Right/6(SLC Tune In)
  Full Mixing Matrix_Center Surround/3(SLC_NTF_done) -> Merge NTF_done/2(SLC_NTF_done_CS)
  Fade Inputs/4(triggerRight) -> Full Mixing Matrix_Right/7(Fade Request Trigger)
  Merge NTF_done/1(SLC_NTF_done) -> SLC_NTF_done/1
  FrontFadeGain/1 -> Fade Inputs/1(FrontGain)
  Split NTF_check_done/3(fcncall_Right()) -> Full Mixing Matrix_Right/5(SLC_NTF_check_done)
  Fade Tuning/1(Fade Tune Out) -> Full Mixing Matrix_Left/10(Fade Tune In), Full Mixing Matrix_Center Surround/10(Fade Tune In), Full Mixing Matrix_Right/10(Fade Tune In)
  Full Mixing Matrix_Right/1(Output) -> [Right_Output]
  DR-FDP Output/1 -> Input Organizer/2(DR-FDP O/P)
  Function-Call Split1/3 -> Full Mixing Matrix_Right/3(SLC Request Trigger)
  CAE/1 -> [CAE_Enable]
  Full Mixing Matrix_Center Surround/2(MS Mixing Gains) -> [MS_MixCoeff]
  Input Organizer/2(CS Channel Inputs) -> [CS_Input], Full Mixing Matrix_Center Surround/1(Audio Channel Inputs)
  [C_Output] -> CS Processing/1(COut)
  CS Processing/1(CSOut) -> [CS_Output]
  [MS_MixCoeff] -> CS Processing/3(MixCoeff)
  [CS_Input] -> CS Processing/2(ChanIn)

== system MedusaPremix/Premix/Fade Inputs ==
  FrontGain : Inport
  BackGain : Inport  Port=2
  Abs : Abs  SaturateOnIntegerOverflow=off
  Abs1 : Abs  SaturateOnIntegerOverflow=off
  Add : Sum
  Delay : Delay  DelayLength=1  InitialCondition=0
  Delay1 : Delay  DelayLength=1  InitialCondition=0
  Fade_Trigger_Generation : MATLAB Function  TreatAsAtomicUnit=on
  Subtract1 : Sum  Inputs=-+
  Subtract2 : Sum  Inputs=-+
  triggerLeft : Outport  VectorParamsAs1DForOutWhenUnconnected=off
  triggerCS : Outport  Port=2  VectorParamsAs1DForOutWhenUnconnected=off
  triggerRight : Outport  Port=3  VectorParamsAs1DForOutWhenUnconnected=off
  FrontFadeGain : Outport  Port=4  VectorParamsAs1DForOutWhenUnconnected=off
  BackFadeGain : Outport  Port=5  VectorParamsAs1DForOutWhenUnconnected=off
  wires:
  Fade_Trigger_Generation/1(fadeTrigger_Left()) -> triggerLeft/1
  Fade_Trigger_Generation/3(fadeTrigger_Right()) -> triggerRight/1
  Add/1 -> Fade_Trigger_Generation/1(gainDifference)
  Fade_Trigger_Generation/2(fadeTrigger_CS()) -> triggerCS/1
  Delay1/1 -> Subtract2/1
  Delay/1 -> Subtract1/1
  FrontGain/1 -> Delay/1, FrontFadeGain/1, Subtract1/2
  Subtract1/1 -> Abs/1
  Subtract2/1 -> Abs1/1
  Abs/1 -> Add/1
  Abs1/1 -> Add/2
  BackGain/1 -> Delay1/1, Subtract2/2, BackFadeGain/1

== system MedusaPremix/Premix/Fade Tuning ==
  Backward Downmix Max : Subsystem  Description=This is the fraction of downmixing that occurs when 100% fade (back) is reached.
  Backward Downmix Threshold : Subsystem  Description=This is the fraction of fade (back) at which downmixing of premix coefficients starts.
  Downmix Weights CS : Subsystem  Description=These are the mixing weights at fader extreme when downmix_max is set to 1.
  Downmix Weights Left : Subsystem  Description=These are the mixing weights at fader extreme when downmix_max is set to 1.
  Downmix Weights Right : Subsystem  Description=These are the mixing weights at fader extreme when downmix_max is set to 1.
  Forward Downmix Threshold : Subsystem  Description=This is the fraction of fade (front) at which downmixing of premix coefficients starts.
  Foward Downmix Max : Subsystem  Description=This is the fraction of downmixing that occurs when 100% fade (front) is reached.
  Bus Element Out : Outport  VectorParamsAs1DForOutWhenUnconnected=off  PortName=Fade Tune Out  Element=Forward Downmix Threshold
  Bus Element Out1 : Outport  VectorParamsAs1DForOutWhenUnconnected=off  PortName=Fade Tune Out  Element=Forward Downmix Max
  Bus Element Out2 : Outport  VectorParamsAs1DForOutWhenUnconnected=off  PortName=Fade Tune Out  Element=Backward Downmix Threshold
  Bus Element Out3 : Outport  VectorParamsAs1DForOutWhenUnconnected=off  PortName=Fade Tune Out  Element=Backward Downmix Max
  Bus Element Out4 : Outport  VectorParamsAs1DForOutWhenUnconnected=off  PortName=Fade Tune Out  Element=Downmix Weights Left
  Bus Element Out5 : Outport  VectorParamsAs1DForOutWhenUnconnected=off  PortName=Fade Tune Out  Element=Downmix Weights CS
  Bus Element Out6 : Outport  VectorParamsAs1DForOutWhenUnconnected=off  PortName=Fade Tune Out  Element=Downmix Weights Right
  wires:
  Forward Downmix Threshold/1(Out1) -> Bus Element Out/1
  Foward Downmix Max/1(Out1) -> Bus Element Out1/1
  Backward Downmix Max/1(Out1) -> Bus Element Out3/1
  Backward Downmix Threshold/1(Out1) -> Bus Element Out2/1
  Downmix Weights Left/1(Out1) -> Bus Element Out4/1
  Downmix Weights CS/1(Out1) -> Bus Element Out5/1
  Downmix Weights Right/1(Out1) -> Bus Element Out6/1
